simulink model "parallel"  (R2015b)
settings: Solver=FixedStepDiscrete  SolverMode=SingleTasking  StartTime=0.0  StopTime=600e-6  RelTol=1e-3
values from neighbouring files (symbols this model uses):
  b = ['00';'02';'04';'06';'08';'0a';'0c';'0e';'10';'12';'14';'16';'18';'1a';'1c';'1e';'20';'22';'24';'26';'28';'2a';'2c';'2e';'30';'32';'34';'36';'38';'3a';'3c';'3e';'40';'42';'44';'46';'48';'4a';'4c';'4e';'50';'52';'54';'56';'58';'5a';'5c';'5e';'60';'62';'64';'66';'68';'6a';'6c';'6e';'70';'72';'74';'76';'78';'7a';'7c';'7e';'80';'82';'84';'86';'88';'8a';'8c';'8e';'90';'92';'94';'96';'98';'9a';'9c';'9e' ...(+881 chars)    [parallelpipe_tb.m]
  input_sample_rate = 1.0E06    (= 1000000)    [parallelpipe_tb.m]
undefined symbols (not defined in the file or in its folder): a
libraries: shlslibv1 x6037
(part 2 of 40)

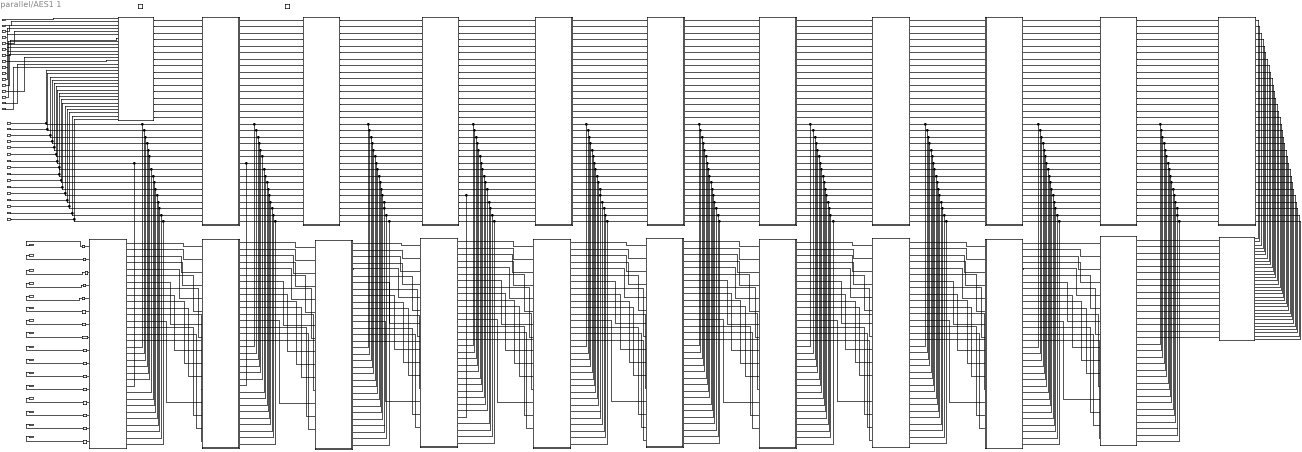
== system parallel/AES1 1 ==
  In1 : Inport
  In2 : Inport  Port=2
  In3 : Inport  Port=3
  In4 : Inport  Port=4
  In5 : Inport  Port=5
  In6 : Inport  Port=6
  In7 : Inport  Port=7
  In8 : Inport  Port=8
  In9 : Inport  Port=9
  In10 : Inport  Port=10
  In11 : Inport  Port=11
  In12 : Inport  Port=12
  In13 : Inport  Port=13
  In14 : Inport  Port=14
  In15 : Inport  Port=15
  In16 : Inport  Port=16
  In17 : Inport  Port=17
  In18 : Inport  Port=18
  In19 : Inport  Port=19
  In20 : Inport  Port=20
  In21 : Inport  Port=21
  In22 : Inport  Port=22
  In23 : Inport  Port=23
  In24 : Inport  Port=24
  In25 : Inport  Port=25
  In26 : Inport  Port=26
  In27 : Inport  Port=27
  In28 : Inport  Port=28
  In29 : Inport  Port=29
  In30 : Inport  Port=30
  In31 : Inport  Port=31
  In32 : Inport  Port=32
  Port Out{32..47} (16 alike) : shlslibv1/Ports & Subsystems/Port Out  syn_capture=on  syn_register=on  synBlockType=port  synLatency=1  synBlockId=1
  Round1 : Subsystem
  Round10 : Subsystem
  Round11 : Subsystem
  Round12 : Subsystem
  Round13 : Subsystem
  Round14 : Subsystem
  Round15 : Subsystem
  Round16 : Subsystem
  Round17 : Subsystem
  Round18 : Subsystem
  Round19 : Subsystem
  Round2 : Subsystem
  Round20 : Subsystem
  Round3 : Subsystem
  Round4 : Subsystem
  Round5 : Subsystem
  Round6 : Subsystem
  Round7 : Subsystem
  Round8 : Subsystem
  Round9 : Subsystem
  SHLSTool1 : shlslibv1/SHLSTool  synBlockType=tool  syn_dsp_mode=FPGA
  Subsystem : Subsystem
  Subsystem2 : Subsystem
  Test Vector Capture : shlslibv1/Ports & Subsystems/Test Vector Capture  syn_capture_mode=on
  Out1 : Outport
  Out2 : Outport  Port=2
  Out3 : Outport  Port=3
  Out4 : Outport  Port=4
  Out5 : Outport  Port=5
  Out6 : Outport  Port=6
  Out7 : Outport  Port=7
  Out8 : Outport  Port=8
  Out9 : Outport  Port=9
  Out10 : Outport  Port=10
  Out11 : Outport  Port=11
  Out12 : Outport  Port=12
  Out13 : Outport  Port=13
  Out14 : Outport  Port=14
  Out15 : Outport  Port=15
  Out16 : Outport  Port=16
  wires:
  Round1/1(Out1) -> Round2/1(In1)
  Round1/2(Out2) -> Round2/2(In2)
  Round1/3(Out3) -> Round2/3(In3)
  Round1/4(Out4) -> Round2/4(In4)
  Round1/5(Out5) -> Round2/5(In5)
  Round1/6(Out6) -> Round2/6(In6)
  Round1/7(Out7) -> Round2/7(In7)
  Round1/8(Out8) -> Round2/8(In8)
  Round1/9(Out9) -> Round2/9(In9)
  Round1/10(Out10) -> Round2/10(In10)
  Round1/11(Out11) -> Round2/11(In11)
  Round1/12(Out12) -> Round2/12(In12)
  Round1/13(Out13) -> Round2/13(In13)
  Round1/14(Out14) -> Round2/14(In14)
  Round1/15(Out15) -> Round2/15(In15)
  Round1/16(Out16) -> Round2/16(In16)
  Round2/2(Out2) -> Round4/2(In2)
  Round2/3(Out3) -> Round4/3(In3)
  Round2/4(Out4) -> Round4/4(In4)
  Round2/5(Out5) -> Round4/5(In5)
  Round2/6(Out6) -> Round4/6(In6)
  Round2/7(Out7) -> Round4/7(In7)
  Round2/8(Out8) -> Round4/8(In8)
  Round2/9(Out9) -> Round4/9(In9)
  Round2/10(Out10) -> Round4/10(In10)
  Round2/11(Out11) -> Round4/11(In11)
  Round2/12(Out12) -> Round4/12(In12)
  Round2/13(Out13) -> Round4/13(In13)
  Round2/14(Out14) -> Round4/14(In14)
  Round2/15(Out15) -> Round4/15(In15)
  Round2/16(Out16) -> Round4/16(In16)
  Round2/1(Out1) -> Round4/1(In1)
  Round4/1(Out1) -> Round5/1(In1)
  Round4/2(Out2) -> Round5/2(In2)
  Round3/2(Out2) -> Round6/2(In2)
  Round4/3(Out3) -> Round5/3(In3)
  Round4/4(Out4) -> Round5/4(In4)
  Round4/5(Out5) -> Round5/5(In5)
  Round4/6(Out6) -> Round5/6(In6)
  Round4/7(Out7) -> Round5/7(In7)
  Round4/8(Out8) -> Round5/8(In8)
  Round4/9(Out9) -> Round5/9(In9)
  Round4/10(Out10) -> Round5/10(In10)
  Round4/11(Out11) -> Round5/11(In11)
  Round4/12(Out12) -> Round5/12(In12)
  Round4/13(Out13) -> Round5/13(In13)
  Round4/14(Out14) -> Round5/14(In14)
  Round4/15(Out15) -> Round5/15(In15)
  Round4/16(Out16) -> Round5/16(In16)
  Round5/2(Out2) -> Round3/2(In2)
  Round5/3(Out3) -> Round3/3(In3)
  Round5/4(Out4) -> Round3/4(In4)
  Round5/5(Out5) -> Round3/5(In5)
  Round5/6(Out6) -> Round3/6(In6)
  Round5/7(Out7) -> Round3/7(In7)
  Round5/8(Out8) -> Round3/8(In8)
  Round5/9(Out9) -> Round3/9(In9)
  Round5/10(Out10) -> Round3/10(In10)
  Round5/11(Out11) -> Round3/11(In11)
  Round5/12(Out12) -> Round3/12(In12)
  Round5/13(Out13) -> Round3/13(In13)
  Round5/14(Out14) -> Round3/14(In14)
  Round5/15(Out15) -> Round3/15(In15)
  Round5/16(Out16) -> Round3/16(In16)
  Round5/1(Out1) -> Round3/1(In1)
  Round3/1(Out1) -> Round6/1(In1)
  Round9/3(Out3) -> Round10/3(In3)
  Round9/2(Out2) -> Round10/2(In2)
  Round3/3(Out3) -> Round6/3(In3)
  Round3/4(Out4) -> Round6/4(In4)
  Round3/5(Out5) -> Round6/5(In5)
  Round3/6(Out6) -> Round6/6(In6)
  Round3/7(Out7) -> Round6/7(In7)
  Round3/8(Out8) -> Round6/8(In8)
  Round3/9(Out9) -> Round6/9(In9)
  Round3/10(Out10) -> Round6/10(In10)
  Round3/11(Out11) -> Round6/11(In11)
  Round3/12(Out12) -> Round6/12(In12)
  Round3/13(Out13) -> Round6/13(In13)
  Round3/14(Out14) -> Round6/14(In14)
  Round3/15(Out15) -> Round6/15(In15)
  Round3/16(Out16) -> Round6/16(In16)
  Round6/1(Out1) -> Round7/1(In1)
  Round6/2(Out2) -> Round7/2(In2)
  Round6/3(Out3) -> Round7/3(In3)
  Round6/4(Out4) -> Round7/4(In4)
  Round6/5(Out5) -> Round7/5(In5)
  Round6/6(Out6) -> Round7/6(In6)
  Round6/7(Out7) -> Round7/7(In7)
  Round6/8(Out8) -> Round7/8(In8)
  Round6/9(Out9) -> Round7/9(In9)
  Round6/10(Out10) -> Round7/10(In10)
  Round6/11(Out11) -> Round7/11(In11)
  Round6/12(Out12) -> Round7/12(In12)
  Round6/13(Out13) -> Round7/13(In13)
  Round6/14(Out14) -> Round7/14(In14)
  Round6/15(Out15) -> Round7/15(In15)
  Round6/16(Out16) -> Round7/16(In16)
  Round7/1(Out1) -> Round8/1(In1)
  Round7/2(Out2) -> Round8/2(In2)
  Round7/3(Out3) -> Round8/3(In3)
  Round7/4(Out4) -> Round8/4(In4)
  Round7/5(Out5) -> Round8/5(In5)
  Round7/6(Out6) -> Round8/6(In6)
  Round7/7(Out7) -> Round8/7(In7)
  Round7/8(Out8) -> Round8/8(In8)
  Round7/9(Out9) -> Round8/9(In9)
  Round7/10(Out10) -> Round8/10(In10)
  Round7/11(Out11) -> Round8/11(In11)
  Round7/12(Out12) -> Round8/12(In12)
  Round7/13(Out13) -> Round8/13(In13)
  Round7/14(Out14) -> Round8/14(In14)
  Round7/15(Out15) -> Round8/15(In15)
  Round7/16(Out16) -> Round8/16(In16)
  Round8/1(Out1) -> Round9/1(In1)
  Round8/2(Out2) -> Round9/2(In2)
  Round8/3(Out3) -> Round9/3(In3)
  Round8/4(Out4) -> Round9/4(In4)
  Round8/5(Out5) -> Round9/5(In5)
  Round8/6(Out6) -> Round9/6(In6)
  Round8/7(Out7) -> Round9/7(In7)
  Round8/8(Out8) -> Round9/8(In8)
  Round8/9(Out9) -> Round9/9(In9)
  Round8/10(Out10) -> Round9/10(In10)
  Round8/11(Out11) -> Round9/11(In11)
  Round8/12(Out12) -> Round9/12(In12)
  Round8/13(Out13) -> Round9/13(In13)
  Round8/14(Out14) -> Round9/14(In14)
  Round8/15(Out15) -> Round9/15(In15)
  Round8/16(Out16) -> Round9/16(In16)
  Round9/1(Out1) -> Round10/1(In1)
  Round9/21(Out21) -> Round13/21(In21), Round10/21(In21)
  Round9/19(Out19) -> Round13/19(In19), Round10/19(In19)
  Round9/4(Out4) -> Round10/4(In4)
  Round9/5(Out5) -> Round10/5(In5)
  Round9/6(Out6) -> Round10/6(In6)
  Round9/7(Out7) -> Round10/7(In7)
  Round9/8(Out8) -> Round10/8(In8)
  Round9/9(Out9) -> Round10/9(In9)
  Round9/10(Out10) -> Round10/10(In10)
  Round9/11(Out11) -> Round10/11(In11)
  Round9/12(Out12) -> Round10/12(In12)
  Round9/13(Out13) -> Round10/13(In13)
  Round9/14(Out14) -> Round10/14(In14)
  Round9/15(Out15) -> Round10/15(In15)
  Round9/16(Out16) -> Round10/16(In16)
  Subsystem/1(Out1) -> Round1/1(In1)
  Subsystem/2(Out2) -> Round1/2(In2)
  Subsystem/3(Out3) -> Round1/3(In3)
  Subsystem/4(Out4) -> Round1/4(In4)
  Subsystem/5(Out5) -> Round1/5(In5)
  Subsystem/6(Out6) -> Round1/6(In6)
  Subsystem/7(Out7) -> Round1/7(In7)
  Subsystem/8(Out8) -> Round1/8(In8)
  Subsystem/9(Out9) -> Round1/9(In9)
  Subsystem/10(Out10) -> Round1/10(In10)
  Subsystem/11(Out11) -> Round1/11(In11)
  Subsystem/12(Out12) -> Round1/12(In12)
  Subsystem/13(Out13) -> Round1/13(In13)
  Subsystem/14(Out14) -> Round1/14(In14)
  Subsystem/15(Out15) -> Round1/15(In15)
  Subsystem/16(Out16) -> Round1/16(In16)
  In1/1 -> Subsystem/1(In1)
  In2/1 -> Subsystem/2(In2)
  In3/1 -> Subsystem/3(In3)
  In4/1 -> Subsystem/4(In4)
  In5/1 -> Subsystem/5(In5)
  In6/1 -> Subsystem/6(In6)
  In7/1 -> Subsystem/7(In7)
  In8/1 -> Subsystem/8(In8)
  In9/1 -> Subsystem/9(In9)
  In10/1 -> Subsystem/10(In10)
  In11/1 -> Subsystem/11(In11)
  In12/1 -> Subsystem/12(In12)
  In13/1 -> Subsystem/13(In13)
  In14/1 -> Subsystem/14(In14)
  In15/1 -> Subsystem/15(In15)
  In16/1 -> Subsystem/16(In16)
  Round10/11(Out11) -> Subsystem2/11(In11)
  Round10/13(Out13) -> Subsystem2/13(In13)
  Round10/15(Out15) -> Subsystem2/15(In15)
  Round10/17(Out17) -> Subsystem2/17(In17)
  Round10/19(Out19) -> Subsystem2/19(In19)
  Round10/21(Out21) -> Subsystem2/21(In21)
  Round10/23(Out23) -> Subsystem2/23(In23)
  Round10/27(Out27) -> Subsystem2/27(In27)
  Round10/29(Out29) -> Subsystem2/29(In29)
  Round10/25(Out25) -> Subsystem2/25(In25)
  Round10/2(Out2) -> Subsystem2/2(In2)
  Round10/12(Out12) -> Subsystem2/12(In12)
  Round10/14(Out14) -> Subsystem2/14(In14)
  Round10/16(Out16) -> Subsystem2/16(In16)
  Round10/18(Out18) -> Subsystem2/18(In18)
  Round10/20(Out20) -> Subsystem2/20(In20)
  Round10/22(Out22) -> Subsystem2/22(In22)
  Round10/24(Out24) -> Subsystem2/24(In24)
  Round10/28(Out28) -> Subsystem2/28(In28)
  Round10/30(Out30) -> Subsystem2/30(In30)
  Round10/26(Out26) -> Subsystem2/26(In26)
  Round10/1(Out1) -> Subsystem2/1(In1)
  Round10/3(Out3) -> Subsystem2/3(In3)
  Round10/4(Out4) -> Subsystem2/4(In4)
  Round10/5(Out5) -> Subsystem2/5(In5)
  Round10/6(Out6) -> Subsystem2/6(In6)
  Round10/7(Out7) -> Subsystem2/7(In7)
  Round10/8(Out8) -> Subsystem2/8(In8)
  Round10/9(Out9) -> Subsystem2/9(In9)
  Round10/10(Out10) -> Subsystem2/10(In10)
  Round10/31(Out31) -> Subsystem2/31(In31)
  Round10/32(Out32) -> Subsystem2/32(In32)
  Subsystem2/1(Out1) -> Round13/1(In1)
  Subsystem2/2(Out2) -> Round13/2(In2)
  Subsystem2/3(Out3) -> Round13/3(In3)
  Subsystem2/4(Out4) -> Round13/4(In4)
  Subsystem2/5(Out5) -> Round13/5(In5)
  Subsystem2/6(Out6) -> Round13/6(In6)
  Subsystem2/7(Out7) -> Round13/7(In7)
  Subsystem2/8(Out8) -> Round13/8(In8)
  Subsystem2/9(Out9) -> Round13/9(In9)
  Subsystem2/10(Out10) -> Round13/10(In10)
  Subsystem2/11(Out11) -> Round13/11(In11)
  Subsystem2/12(Out12) -> Round13/12(In12)
  Subsystem2/13(Out13) -> Round13/13(In13)
  Subsystem2/14(Out14) -> Round13/14(In14)
  Subsystem2/15(Out15) -> Round13/15(In15)
  Subsystem2/16(Out16) -> Round13/16(In16)
  Round9/17(Out17) -> Round13/17(In17), Round10/17(In17)
  Round1/17(Out17) -> Round19/17(In17), Round2/17(In17)
  Round1/19(Out19) -> Round19/19(In19), Round2/19(In19)
  Round1/21(Out21) -> Round19/21(In21), Round2/21(In21)
  Round1/23(Out23) -> Round2/23(In23), Round19/23(In23)
  Round9/23(Out23) -> Round13/23(In23), Round10/23(In23)
  Round9/27(Out27) -> Round13/27(In27), Round10/27(In27)
  Round9/29(Out29) -> Round13/29(In29), Round10/29(In29)
  Round9/25(Out25) -> Round13/25(In25), Round10/25(In25)
  Round9/18(Out18) -> Round13/18(In18), Round10/18(In18)
  Round9/20(Out20) -> Round13/20(In20), Round10/20(In20)
  Round9/22(Out22) -> Round13/22(In22), Round10/22(In22)
  Round9/24(Out24) -> Round13/24(In24), Round10/24(In24)
  Round9/28(Out28) -> Round13/28(In28), Round10/28(In28)
  Round9/30(Out30) -> Round13/30(In30), Round10/30(In30)
  Round9/26(Out26) -> Round13/26(In26), Round10/26(In26)
  Round9/31(Out31) -> Round13/31(In31), Round10/31(In31)
  Round9/32(Out32) -> Round13/32(In32), Round10/32(In32)
  Port Out32/1 -> Out1/1
  Port Out33/1 -> Out2/1
  Port Out36/1 -> Out3/1
  Port Out42/1 -> Out4/1
  Port Out43/1 -> Out5/1
  Port Out44/1 -> Out6/1
  Port Out45/1 -> Out7/1
  Port Out46/1 -> Out8/1
  Port Out47/1 -> Out10/1
  Port Out34/1 -> Out11/1
  Port Out35/1 -> Out12/1
  Port Out37/1 -> Out13/1
  Port Out38/1 -> Out14/1
  Port Out39/1 -> Out15/1
  Port Out40/1 -> Out16/1
  Round13/1(Out1) -> Round11/1(In1)
  Round8/17(Out17) -> Round11/17(In17), Round9/17(In17)
  Round8/19(Out19) -> Round11/19(In19), Round9/19(In19)
  Round8/21(Out21) -> Round11/21(In21), Round9/21(In21)
  Round8/23(Out23) -> Round11/23(In23), Round9/23(In23)
  Round8/27(Out27) -> Round11/27(In27), Round9/27(In27)
  Round8/29(Out29) -> Round11/29(In29), Round9/29(In29)
  Round8/25(Out25) -> Round11/25(In25), Round9/25(In25)
  Round8/18(Out18) -> Round11/18(In18), Round9/18(In18)
  Round8/20(Out20) -> Round11/20(In20), Round9/20(In20)
  Round8/22(Out22) -> Round11/22(In22), Round9/22(In22)
  Round8/24(Out24) -> Round11/24(In24), Round9/24(In24)
  Round8/28(Out28) -> Round11/28(In28), Round9/28(In28)
  Round8/30(Out30) -> Round11/30(In30), Round9/30(In30)
  Round8/26(Out26) -> Round11/26(In26), Round9/26(In26)
  Round8/31(Out31) -> Round11/31(In31), Round9/31(In31)
  Round8/32(Out32) -> Round11/32(In32), Round9/32(In32)
  Round13/2(Out2) -> Round11/2(In2)
  Round13/3(Out3) -> Round11/3(In3)
  Round13/4(Out4) -> Round11/4(In4)
  Round13/5(Out5) -> Round11/5(In5)
  Round13/6(Out6) -> Round11/6(In6)
  Round13/7(Out7) -> Round11/7(In7)
  Round13/8(Out8) -> Round11/8(In8)
  Round13/9(Out9) -> Round11/9(In9)
  Round13/10(Out10) -> Round11/10(In10)
  Round13/11(Out11) -> Round11/11(In11)
  Round13/12(Out12) -> Round11/12(In12)
  Round13/13(Out13) -> Round11/13(In13)
  Round13/14(Out14) -> Round11/14(In14)
  Round13/15(Out15) -> Round11/15(In15)
  Round13/16(Out16) -> Round11/16(In16)
  Port Out41/1 -> Out9/1
  Round11/1(Out1) -> Round12/1(In1)
  Round7/17(Out17) -> Round12/17(In17), Round8/17(In17)
  Round7/19(Out19) -> Round12/19(In19), Round8/19(In19)
  Round7/21(Out21) -> Round12/21(In21), Round8/21(In21)
  Round7/23(Out23) -> Round12/23(In23), Round8/23(In23)
  Round7/27(Out27) -> Round12/27(In27), Round8/27(In27)
  Round7/29(Out29) -> Round12/29(In29), Round8/29(In29)
  Round7/25(Out25) -> Round12/25(In25), Round8/25(In25)
  Round7/18(Out18) -> Round12/18(In18), Round8/18(In18)
  Round7/20(Out20) -> Round12/20(In20), Round8/20(In20)
  Round7/22(Out22) -> Round12/22(In22), Round8/22(In22)
  Round7/24(Out24) -> Round12/24(In24), Round8/24(In24)
  Round7/28(Out28) -> Round12/28(In28), Round8/28(In28)
  Round7/30(Out30) -> Round12/30(In30), Round8/30(In30)
  Round7/26(Out26) -> Round12/26(In26), Round8/26(In26)
  Round7/31(Out31) -> Round12/31(In31), Round8/31(In31)
  Round7/32(Out32) -> Round12/32(In32), Round8/32(In32)
  Round11/2(Out2) -> Round12/2(In2)
  Round11/3(Out3) -> Round12/3(In3)
  Round11/4(Out4) -> Round12/4(In4)
  Round11/5(Out5) -> Round12/5(In5)
  Round11/6(Out6) -> Round12/6(In6)
  Round11/7(Out7) -> Round12/7(In7)
  Round11/8(Out8) -> Round12/8(In8)
  Round11/9(Out9) -> Round12/9(In9)
  Round11/10(Out10) -> Round12/10(In10)
  Round11/11(Out11) -> Round12/11(In11)
  Round11/12(Out12) -> Round12/12(In12)
  Round11/13(Out13) -> Round12/13(In13)
  Round11/14(Out14) -> Round12/14(In14)
  Round11/15(Out15) -> Round12/15(In15)
  Round11/16(Out16) -> Round12/16(In16)
  Round12/1(Out1) -> Round14/1(In1)
  Round6/17(Out17) -> Round14/17(In17), Round7/17(In17)
  Round6/19(Out19) -> Round14/19(In19), Round7/19(In19)
  Round6/21(Out21) -> Round14/21(In21), Round7/21(In21)
  Round6/23(Out23) -> Round14/23(In23), Round7/23(In23)
  Round6/27(Out27) -> Round14/27(In27), Round7/27(In27)
  Round6/29(Out29) -> Round14/29(In29), Round7/29(In29)
  Round6/25(Out25) -> Round14/25(In25), Round7/25(In25)
  Round6/18(Out18) -> Round14/18(In18), Round7/18(In18)
  Round6/20(Out20) -> Round14/20(In20), Round7/20(In20)
  Round6/22(Out22) -> Round14/22(In22), Round7/22(In22)
  Round6/24(Out24) -> Round14/24(In24), Round7/24(In24)
  Round6/28(Out28) -> Round14/28(In28), Round7/28(In28)
  Round6/30(Out30) -> Round14/30(In30), Round7/30(In30)
  Round6/26(Out26) -> Round14/26(In26), Round7/26(In26)
  Round6/31(Out31) -> Round14/31(In31), Round7/31(In31)
  Round6/32(Out32) -> Round14/32(In32), Round7/32(In32)
  Round12/2(Out2) -> Round14/2(In2)
  Round12/3(Out3) -> Round14/3(In3)
  Round12/4(Out4) -> Round14/4(In4)
  Round12/5(Out5) -> Round14/5(In5)
  Round12/6(Out6) -> Round14/6(In6)
  Round12/7(Out7) -> Round14/7(In7)
  Round12/8(Out8) -> Round14/8(In8)
  Round12/9(Out9) -> Round14/9(In9)
  Round12/10(Out10) -> Round14/10(In10)
  Round12/11(Out11) -> Round14/11(In11)
  Round12/12(Out12) -> Round14/12(In12)
  Round12/13(Out13) -> Round14/13(In13)
  Round12/14(Out14) -> Round14/14(In14)
  Round12/15(Out15) -> Round14/15(In15)
  Round12/16(Out16) -> Round14/16(In16)
  Round14/1(Out1) -> Round15/1(In1)
  Round3/17(Out17) -> Round15/17(In17), Round6/17(In17)
  Round3/19(Out19) -> Round15/19(In19), Round6/19(In19)
  Round3/21(Out21) -> Round15/21(In21), Round6/21(In21)
  Round3/23(Out23) -> Round15/23(In23), Round6/23(In23)
  Round3/27(Out27) -> Round15/27(In27), Round6/27(In27)
  Round3/29(Out29) -> Round15/29(In29), Round6/29(In29)
  Round3/25(Out25) -> Round15/25(In25), Round6/25(In25)
  Round3/18(Out18) -> Round15/18(In18), Round6/18(In18)
  Round3/20(Out20) -> Round15/20(In20), Round6/20(In20)
  Round3/22(Out22) -> Round15/22(In22), Round6/22(In22)
  Round3/24(Out24) -> Round15/24(In24), Round6/24(In24)
  Round3/28(Out28) -> Round15/28(In28), Round6/28(In28)
  Round3/30(Out30) -> Round15/30(In30), Round6/30(In30)
  Round3/26(Out26) -> Round15/26(In26), Round6/26(In26)
  Round3/31(Out31) -> Round15/31(In31), Round6/31(In31)
  Round3/32(Out32) -> Round15/32(In32), Round6/32(In32)
  Round14/2(Out2) -> Round15/2(In2)
  Round14/3(Out3) -> Round15/3(In3)
  Round14/4(Out4) -> Round15/4(In4)
  Round14/5(Out5) -> Round15/5(In5)
  Round14/6(Out6) -> Round15/6(In6)
  Round14/7(Out7) -> Round15/7(In7)
  Round14/8(Out8) -> Round15/8(In8)
  Round14/9(Out9) -> Round15/9(In9)
  Round14/10(Out10) -> Round15/10(In10)
  Round14/11(Out11) -> Round15/11(In11)
  Round14/12(Out12) -> Round15/12(In12)
  Round14/13(Out13) -> Round15/13(In13)
  Round14/14(Out14) -> Round15/14(In14)
  Round14/15(Out15) -> Round15/15(In15)
  Round14/16(Out16) -> Round15/16(In16)
  Round15/1(Out1) -> Round16/1(In1)
  Round5/17(Out17) -> Round16/17(In17), Round3/17(In17)
  Round5/19(Out19) -> Round16/19(In19), Round3/19(In19)
  Round5/21(Out21) -> Round16/21(In21), Round3/21(In21)
  Round5/23(Out23) -> Round16/23(In23), Round3/23(In23)
  Round5/27(Out27) -> Round16/27(In27), Round3/27(In27)
  Round5/29(Out29) -> Round16/29(In29), Round3/29(In29)
  Round5/25(Out25) -> Round16/25(In25), Round3/25(In25)
  Round5/18(Out18) -> Round16/18(In18), Round3/18(In18)
  Round5/20(Out20) -> Round16/20(In20), Round3/20(In20)
  Round5/22(Out22) -> Round16/22(In22), Round3/22(In22)
  Round5/24(Out24) -> Round16/24(In24), Round3/24(In24)
  Round5/28(Out28) -> Round16/28(In28), Round3/28(In28)
  Round5/30(Out30) -> Round16/30(In30), Round3/30(In30)
  Round5/26(Out26) -> Round16/26(In26), Round3/26(In26)
  Round5/31(Out31) -> Round16/31(In31), Round3/31(In31)
  Round5/32(Out32) -> Round16/32(In32), Round3/32(In32)
  Round15/2(Out2) -> Round16/2(In2)
  Round15/3(Out3) -> Round16/3(In3)
  Round15/4(Out4) -> Round16/4(In4)
  Round15/5(Out5) -> Round16/5(In5)
  Round15/6(Out6) -> Round16/6(In6)
  Round15/7(Out7) -> Round16/7(In7)
  Round15/8(Out8) -> Round16/8(In8)
  Round15/9(Out9) -> Round16/9(In9)
  Round15/10(Out10) -> Round16/10(In10)
  Round15/11(Out11) -> Round16/11(In11)
  Round15/12(Out12) -> Round16/12(In12)
  Round15/13(Out13) -> Round16/13(In13)
  Round15/14(Out14) -> Round16/14(In14)
  Round15/15(Out15) -> Round16/15(In15)
  Round15/16(Out16) -> Round16/16(In16)
  Round16/1(Out1) -> Round17/1(In1)
  Round4/17(Out17) -> Round17/17(In17), Round5/17(In17)
  Round4/19(Out19) -> Round17/19(In19), Round5/19(In19)
  Round4/21(Out21) -> Round17/21(In21), Round5/21(In21)
  Round4/23(Out23) -> Round17/23(In23), Round5/23(In23)
  Round4/27(Out27) -> Round17/27(In27), Round5/27(In27)
  Round4/29(Out29) -> Round17/29(In29), Round5/29(In29)
  Round4/25(Out25) -> Round17/25(In25), Round5/25(In25)
  Round4/18(Out18) -> Round17/18(In18), Round5/18(In18)
  Round4/20(Out20) -> Round17/20(In20), Round5/20(In20)
  Round4/22(Out22) -> Round17/22(In22), Round5/22(In22)
  Round4/24(Out24) -> Round17/24(In24), Round5/24(In24)
  Round4/28(Out28) -> Round5/28(In28), Round17/28(In28)
  Round4/30(Out30) -> Round17/30(In30), Round5/30(In30)
  Round4/26(Out26) -> Round17/26(In26), Round5/26(In26)
  Round4/31(Out31) -> Round17/31(In31), Round5/31(In31)
  Round4/32(Out32) -> Round17/32(In32), Round5/32(In32)
  Round16/2(Out2) -> Round17/2(In2)
  Round16/3(Out3) -> Round17/3(In3)
  Round16/4(Out4) -> Round17/4(In4)
  Round16/5(Out5) -> Round17/5(In5)
  Round16/6(Out6) -> Round17/6(In6)
  Round16/7(Out7) -> Round17/7(In7)
  Round16/8(Out8) -> Round17/8(In8)
  Round16/9(Out9) -> Round17/9(In9)
  Round16/10(Out10) -> Round17/10(In10)
  Round16/11(Out11) -> Round17/11(In11)
  Round16/12(Out12) -> Round17/12(In12)
  Round16/13(Out13) -> Round17/13(In13)
  Round16/14(Out14) -> Round17/14(In14)
  Round16/15(Out15) -> Round17/15(In15)
  Round16/16(Out16) -> Round17/16(In16)
  Round17/1(Out1) -> Round18/1(In1)
  Round2/17(Out17) -> Round18/17(In17), Round4/17(In17)
  Round2/19(Out19) -> Round18/19(In19), Round4/19(In19)
  Round2/21(Out21) -> Round18/21(In21), Round4/21(In21)
  Round2/23(Out23) -> Round18/23(In23), Round4/23(In23)
  Round2/27(Out27) -> Round18/27(In27), Round4/27(In27)
  Round2/29(Out29) -> Round18/29(In29), Round4/29(In29)
  Round2/25(Out25) -> Round18/25(In25), Round4/25(In25)
  Round2/18(Out18) -> Round18/18(In18), Round4/18(In18)
  Round2/20(Out20) -> Round18/20(In20), Round4/20(In20)
  Round2/22(Out22) -> Round18/22(In22), Round4/22(In22)
  Round2/24(Out24) -> Round18/24(In24), Round4/24(In24)
  Round2/28(Out28) -> Round18/28(In28), Round4/28(In28)
  Round2/30(Out30) -> Round4/30(In30), Round18/30(In30)
  Round2/26(Out26) -> Round18/26(In26), Round4/26(In26)
  Round2/31(Out31) -> Round18/31(In31), Round4/31(In31)
  Round2/32(Out32) -> Round18/32(In32), Round4/32(In32)
  Round17/2(Out2) -> Round18/2(In2)
  Round17/3(Out3) -> Round18/3(In3)
  Round17/4(Out4) -> Round18/4(In4)
  Round17/5(Out5) -> Round18/5(In5)
  Round17/6(Out6) -> Round18/6(In6)
  Round17/7(Out7) -> Round18/7(In7)
  Round17/8(Out8) -> Round18/8(In8)
  Round17/9(Out9) -> Round18/9(In9)
  Round17/10(Out10) -> Round18/10(In10)
  Round17/11(Out11) -> Round18/11(In11)
  Round17/12(Out12) -> Round18/12(In12)
  Round17/13(Out13) -> Round18/13(In13)
  Round17/14(Out14) -> Round18/14(In14)
  Round17/15(Out15) -> Round18/15(In15)
  Round17/16(Out16) -> Round18/16(In16)
  Round18/1(Out1) -> Round19/1(In1)
  Round1/27(Out27) -> Round19/27(In27), Round2/27(In27)
  Round1/29(Out29) -> Round19/29(In29), Round2/29(In29)
  Round1/25(Out25) -> Round19/25(In25), Round2/25(In25)
  Round1/18(Out18) -> Round19/18(In18), Round2/18(In18)
  Round1/20(Out20) -> Round19/20(In20), Round2/20(In20)
  Round1/22(Out22) -> Round19/22(In22), Round2/22(In22)
  Round1/24(Out24) -> Round19/24(In24), Round2/24(In24)
  Round1/28(Out28) -> Round19/28(In28), Round2/28(In28)
  Round1/30(Out30) -> Round19/30(In30), Round2/30(In30)
  Round1/26(Out26) -> Round19/26(In26), Round2/26(In26)
  Round1/31(Out31) -> Round19/31(In31), Round2/31(In31)
  Round1/32(Out32) -> Round19/32(In32), Round2/32(In32)
  Round18/2(Out2) -> Round19/2(In2)
  Round18/3(Out3) -> Round19/3(In3)
  Round18/4(Out4) -> Round19/4(In4)
  Round18/5(Out5) -> Round19/5(In5)
  Round18/6(Out6) -> Round19/6(In6)
  Round18/7(Out7) -> Round19/7(In7)
  Round18/8(Out8) -> Round19/8(In8)
  Round18/9(Out9) -> Round19/9(In9)
  Round18/10(Out10) -> Round19/10(In10)
  Round18/11(Out11) -> Round19/11(In11)
  Round18/12(Out12) -> Round19/12(In12)
  Round18/13(Out13) -> Round19/13(In13)
  Round18/14(Out14) -> Round19/14(In14)
  Round18/15(Out15) -> Round19/15(In15)
  Round18/16(Out16) -> Round19/16(In16)
  Round19/1(Out1) -> Round20/1(In1)
  In17/1 -> Round20/17(In17), Round1/17(In17), Subsystem/17(In17)
  In19/1 -> Subsystem/19(In19), Round20/19(In19), Round1/19(In19)
  In21/1 -> Subsystem/21(In21), Round20/21(In21), Round1/21(In21)
  In23/1 -> Subsystem/23(In23), Round20/23(In23), Round1/23(In23)
  In27/1 -> Subsystem/27(In27), Round20/27(In27), Round1/27(In27)
  In29/1 -> Subsystem/29(In29), Round20/29(In29), Round1/29(In29)
  In25/1 -> Subsystem/25(In25), Round20/25(In25), Round1/25(In25)
  In18/1 -> Subsystem/18(In18), Round20/18(In18), Round1/18(In18)
  In20/1 -> Subsystem/20(In20), Round20/20(In20), Round1/20(In20)
  In22/1 -> Subsystem/22(In22), Round20/22(In22), Round1/22(In22)
  In24/1 -> Subsystem/24(In24), Round20/24(In24), Round1/24(In24)
  In28/1 -> Subsystem/28(In28), Round20/28(In28), Round1/28(In28)
  In30/1 -> Subsystem/30(In30), Round20/30(In30), Round1/30(In30)
  In26/1 -> Subsystem/26(In26), Round20/26(In26), Round1/26(In26)
  In31/1 -> Subsystem/31(In31), Round20/31(In31), Round1/31(In31)
  In32/1 -> Subsystem/32(In32), Round20/32(In32), Round1/32(In32)
  Round19/2(Out2) -> Round20/2(In2)
  Round19/3(Out3) -> Round20/3(In3)
  Round19/4(Out4) -> Round20/4(In4)
  Round19/5(Out5) -> Round20/5(In5)
  Round19/6(Out6) -> Round20/6(In6)
  Round19/7(Out7) -> Round20/7(In7)
  Round19/8(Out8) -> Round20/8(In8)
  Round19/9(Out9) -> Round20/9(In9)
  Round19/10(Out10) -> Round20/10(In10)
  Round19/11(Out11) -> Round20/11(In11)
  Round19/12(Out12) -> Round20/12(In12)
  Round19/13(Out13) -> Round20/13(In13)
  Round19/14(Out14) -> Round20/14(In14)
  Round19/15(Out15) -> Round20/15(In15)
  Round19/16(Out16) -> Round20/16(In16)
  Round20/1(Out1) -> Port Out32/1
  Round20/2(Out2) -> Port Out33/1
  Round20/3(Out3) -> Port Out36/1
  Round20/4(Out4) -> Port Out42/1
  Round20/5(Out5) -> Port Out43/1
  Round20/6(Out6) -> Port Out44/1
  Round20/7(Out7) -> Port Out45/1
  Round20/8(Out8) -> Port Out46/1
  Round20/9(Out9) -> Port Out41/1
  Round20/10(Out10) -> Port Out47/1
  Round20/11(Out11) -> Port Out34/1
  Round20/12(Out12) -> Port Out35/1
  Round20/13(Out13) -> Port Out37/1
  Round20/14(Out14) -> Port Out38/1
  Round20/15(Out15) -> Port Out39/1
  Round20/16(Out16) -> Port Out40/1

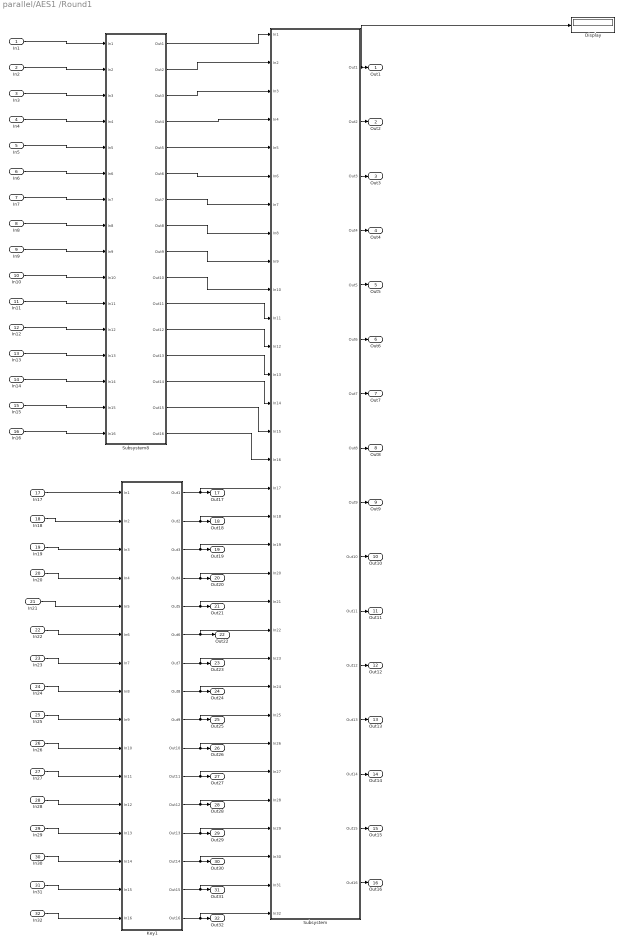
== system parallel/AES1 /Round1 ==
  In1 : Inport
  In2 : Inport  Port=2
  In3 : Inport  Port=3
  In4 : Inport  Port=4
  In5 : Inport  Port=5
  In6 : Inport  Port=6
  In7 : Inport  Port=7
  In8 : Inport  Port=8
  In9 : Inport  Port=9
  In10 : Inport  Port=10
  In11 : Inport  Port=11
  In12 : Inport  Port=12
  In13 : Inport  Port=13
  In14 : Inport  Port=14
  In15 : Inport  Port=15
  In16 : Inport  Port=16
  In17 : Inport  Port=17
  In18 : Inport  Port=18
  In19 : Inport  Port=19
  In20 : Inport  Port=20
  In21 : Inport  Port=21
  In22 : Inport  Port=22
  In23 : Inport  Port=23
  In24 : Inport  Port=24
  In25 : Inport  Port=25
  In26 : Inport  Port=26
  In27 : Inport  Port=27
  In28 : Inport  Port=28
  In29 : Inport  Port=29
  In30 : Inport  Port=30
  In31 : Inport  Port=31
  In32 : Inport  Port=32
  Display : Display
      settings: Format=hex (Stored Integer)
  Key1 : Subsystem
  Subsystem : Subsystem
  Subsystem8 : Subsystem
  Out1 : Outport
  Out2 : Outport  Port=2
  Out3 : Outport  Port=3
  Out4 : Outport  Port=4
  Out5 : Outport  Port=5
  Out6 : Outport  Port=6
  Out7 : Outport  Port=7
  Out8 : Outport  Port=8
  Out9 : Outport  Port=9
  Out10 : Outport  Port=10
  Out11 : Outport  Port=11
  Out12 : Outport  Port=12
  Out13 : Outport  Port=13
  Out14 : Outport  Port=14
  Out15 : Outport  Port=15
  Out16 : Outport  Port=16
  Out17 : Outport  Port=17
  Out18 : Outport  Port=18
  Out19 : Outport  Port=19
  Out20 : Outport  Port=20
  Out21 : Outport  Port=21
  Out22 : Outport  Port=22
  Out23 : Outport  Port=23
  Out24 : Outport  Port=24
  Out25 : Outport  Port=25
  Out26 : Outport  Port=26
  Out27 : Outport  Port=27
  Out28 : Outport  Port=28
  Out29 : Outport  Port=29
  Out30 : Outport  Port=30
  Out31 : Outport  Port=31
  Out32 : Outport  Port=32
  wires:
  Subsystem/14(Out14) -> Out14/1
  Subsystem/6(Out6) -> Out6/1
  Subsystem/13(Out13) -> Out13/1
  Subsystem/10(Out10) -> Out10/1
  Subsystem/5(Out5) -> Out5/1
  Subsystem/7(Out7) -> Out7/1
  Subsystem/8(Out8) -> Out8/1
  Subsystem/3(Out3) -> Out3/1
  Subsystem/2(Out2) -> Out2/1
  Subsystem/16(Out16) -> Out16/1
  Subsystem/9(Out9) -> Out9/1
  Subsystem/12(Out12) -> Out12/1
  Subsystem/15(Out15) -> Out15/1
  Subsystem/4(Out4) -> Out4/1
  Subsystem/11(Out11) -> Out11/1
  In1/1 -> Subsystem8/1(In1)
  In3/1 -> Subsystem8/3(In3)
  In2/1 -> Subsystem8/2(In2)
  In4/1 -> Subsystem8/4(In4)
  In5/1 -> Subsystem8/5(In5)
  In7/1 -> Subsystem8/7(In7)
  In6/1 -> Subsystem8/6(In6)
  In9/1 -> Subsystem8/9(In9)
  In8/1 -> Subsystem8/8(In8)
  In12/1 -> Subsystem8/12(In12)
  In10/1 -> Subsystem8/10(In10)
  In11/1 -> Subsystem8/11(In11)
  In14/1 -> Subsystem8/14(In14)
  In13/1 -> Subsystem8/13(In13)
  In15/1 -> Subsystem8/15(In15)
  In16/1 -> Subsystem8/16(In16)
  Subsystem8/1(Out1) -> Subsystem/1(In1)
  Subsystem8/2(Out2) -> Subsystem/2(In2)
  Subsystem8/4(Out4) -> Subsystem/4(In4)
  Subsystem8/3(Out3) -> Subsystem/3(In3)
  Subsystem8/6(Out6) -> Subsystem/6(In6)
  Subsystem8/5(Out5) -> Subsystem/5(In5)
  Subsystem8/8(Out8) -> Subsystem/8(In8)
  Subsystem8/7(Out7) -> Subsystem/7(In7)
  Subsystem8/10(Out10) -> Subsystem/10(In10)
  Subsystem8/9(Out9) -> Subsystem/9(In9)
  Subsystem8/11(Out11) -> Subsystem/11(In11)
  Subsystem8/12(Out12) -> Subsystem/12(In12)
  Subsystem8/13(Out13) -> Subsystem/13(In13)
  Subsystem8/15(Out15) -> Subsystem/15(In15)
  Subsystem8/14(Out14) -> Subsystem/14(In14)
  Subsystem8/16(Out16) -> Subsystem/16(In16)
  In17/1 -> Key1/1(In1)
  In19/1 -> Key1/3(In3)
  In18/1 -> Key1/2(In2)
  In21/1 -> Key1/5(In5)
  In20/1 -> Key1/4(In4)
  In23/1 -> Key1/7(In7)
  In22/1 -> Key1/6(In6)
  In25/1 -> Key1/9(In9)
  In24/1 -> Key1/8(In8)
  In27/1 -> Key1/11(In11)
  In26/1 -> Key1/10(In10)
  In29/1 -> Key1/13(In13)
  In28/1 -> Key1/12(In12)
  In30/1 -> Key1/14(In14)
  In31/1 -> Key1/15(In15)
  In32/1 -> Key1/16(In16)
  Key1/14(Out14) -> Out30/1, Subsystem/30(In30)
  Key1/6(Out6) -> Out22/1, Subsystem/22(In22)
  Key1/13(Out13) -> Out29/1, Subsystem/29(In29)
  Key1/10(Out10) -> Out26/1, Subsystem/26(In26)
  Key1/5(Out5) -> Out21/1, Subsystem/21(In21)
  Key1/1(Out1) -> Out17/1, Subsystem/17(In17)
  Key1/7(Out7) -> Out23/1, Subsystem/23(In23)
  Key1/8(Out8) -> Out24/1, Subsystem/24(In24)
  Key1/3(Out3) -> Out19/1, Subsystem/19(In19)
  Key1/2(Out2) -> Out18/1, Subsystem/18(In18)
  Key1/16(Out16) -> Out32/1, Subsystem/32(In32)
  Key1/9(Out9) -> Out25/1, Subsystem/25(In25)
  Key1/12(Out12) -> Out28/1, Subsystem/28(In28)
  Key1/15(Out15) -> Out31/1, Subsystem/31(In31)
  Key1/4(Out4) -> Out20/1, Subsystem/20(In20)
  Key1/11(Out11) -> Out27/1, Subsystem/27(In27)
  Subsystem/1(Out1) -> Display/1, Out1/1

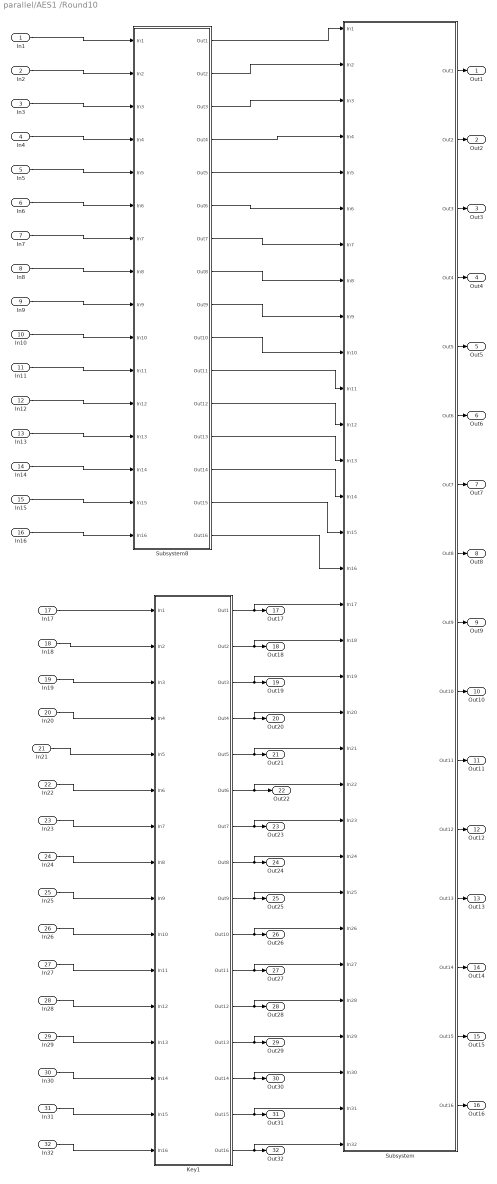
== system parallel/AES1 /Round10 ==
  In1 : Inport
  In2 : Inport  Port=2
  In3 : Inport  Port=3
  In4 : Inport  Port=4
  In5 : Inport  Port=5
  In6 : Inport  Port=6
  In7 : Inport  Port=7
  In8 : Inport  Port=8
  In9 : Inport  Port=9
  In10 : Inport  Port=10
  In11 : Inport  Port=11
  In12 : Inport  Port=12
  In13 : Inport  Port=13
  In14 : Inport  Port=14
  In15 : Inport  Port=15
  In16 : Inport  Port=16
  In17 : Inport  Port=17
  In18 : Inport  Port=18
  In19 : Inport  Port=19
  In20 : Inport  Port=20
  In21 : Inport  Port=21
  In22 : Inport  Port=22
  In23 : Inport  Port=23
  In24 : Inport  Port=24
  In25 : Inport  Port=25
  In26 : Inport  Port=26
  In27 : Inport  Port=27
  In28 : Inport  Port=28
  In29 : Inport  Port=29
  In30 : Inport  Port=30
  In31 : Inport  Port=31
  In32 : Inport  Port=32
  Key1 : Subsystem
  Subsystem : Subsystem
  Subsystem8 : Subsystem
  Out1 : Outport
  Out2 : Outport  Port=2
  Out3 : Outport  Port=3
  Out4 : Outport  Port=4
  Out5 : Outport  Port=5
  Out6 : Outport  Port=6
  Out7 : Outport  Port=7
  Out8 : Outport  Port=8
  Out9 : Outport  Port=9
  Out10 : Outport  Port=10
  Out11 : Outport  Port=11
  Out12 : Outport  Port=12
  Out13 : Outport  Port=13
  Out14 : Outport  Port=14
  Out15 : Outport  Port=15
  Out16 : Outport  Port=16
  Out17 : Outport  Port=17
  Out18 : Outport  Port=18
  Out19 : Outport  Port=19
  Out20 : Outport  Port=20
  Out21 : Outport  Port=21
  Out22 : Outport  Port=22
  Out23 : Outport  Port=23
  Out24 : Outport  Port=24
  Out25 : Outport  Port=25
  Out26 : Outport  Port=26
  Out27 : Outport  Port=27
  Out28 : Outport  Port=28
  Out29 : Outport  Port=29
  Out30 : Outport  Port=30
  Out31 : Outport  Port=31
  Out32 : Outport  Port=32
  wires:
  Subsystem/14(Out14) -> Out14/1
  Subsystem/6(Out6) -> Out6/1
  Subsystem/13(Out13) -> Out13/1
  Subsystem/10(Out10) -> Out10/1
  Subsystem/5(Out5) -> Out5/1
  Subsystem/1(Out1) -> Out1/1
  Subsystem/7(Out7) -> Out7/1
  Subsystem/8(Out8) -> Out8/1
  Subsystem/3(Out3) -> Out3/1
  Subsystem/2(Out2) -> Out2/1
  Subsystem/16(Out16) -> Out16/1
  Subsystem/9(Out9) -> Out9/1
  Subsystem/12(Out12) -> Out12/1
  Subsystem/15(Out15) -> Out15/1
  Subsystem/4(Out4) -> Out4/1
  Subsystem/11(Out11) -> Out11/1
  In1/1 -> Subsystem8/1(In1)
  In3/1 -> Subsystem8/3(In3)
  In2/1 -> Subsystem8/2(In2)
  In4/1 -> Subsystem8/4(In4)
  In5/1 -> Subsystem8/5(In5)
  In7/1 -> Subsystem8/7(In7)
  In6/1 -> Subsystem8/6(In6)
  In9/1 -> Subsystem8/9(In9)
  In8/1 -> Subsystem8/8(In8)
  In12/1 -> Subsystem8/12(In12)
  In10/1 -> Subsystem8/10(In10)
  In11/1 -> Subsystem8/11(In11)
  In14/1 -> Subsystem8/14(In14)
  In13/1 -> Subsystem8/13(In13)
  In15/1 -> Subsystem8/15(In15)
  In16/1 -> Subsystem8/16(In16)
  Subsystem8/1(Out1) -> Subsystem/1(In1)
  Subsystem8/2(Out2) -> Subsystem/2(In2)
  Subsystem8/4(Out4) -> Subsystem/4(In4)
  Subsystem8/3(Out3) -> Subsystem/3(In3)
  Subsystem8/6(Out6) -> Subsystem/6(In6)
  Subsystem8/5(Out5) -> Subsystem/5(In5)
  Subsystem8/8(Out8) -> Subsystem/8(In8)
  Subsystem8/7(Out7) -> Subsystem/7(In7)
  Subsystem8/10(Out10) -> Subsystem/10(In10)
  Subsystem8/9(Out9) -> Subsystem/9(In9)
  Subsystem8/11(Out11) -> Subsystem/11(In11)
  Subsystem8/12(Out12) -> Subsystem/12(In12)
  Subsystem8/13(Out13) -> Subsystem/13(In13)
  Subsystem8/15(Out15) -> Subsystem/15(In15)
  Subsystem8/14(Out14) -> Subsystem/14(In14)
  Subsystem8/16(Out16) -> Subsystem/16(In16)
  In17/1 -> Key1/1(In1)
  In19/1 -> Key1/3(In3)
  In18/1 -> Key1/2(In2)
  In21/1 -> Key1/5(In5)
  In20/1 -> Key1/4(In4)
  In23/1 -> Key1/7(In7)
  In22/1 -> Key1/6(In6)
  In25/1 -> Key1/9(In9)
  In24/1 -> Key1/8(In8)
  In27/1 -> Key1/11(In11)
  In26/1 -> Key1/10(In10)
  In29/1 -> Key1/13(In13)
  In28/1 -> Key1/12(In12)
  In30/1 -> Key1/14(In14)
  In31/1 -> Key1/15(In15)
  In32/1 -> Key1/16(In16)
  Key1/14(Out14) -> Out30/1, Subsystem/30(In30)
  Key1/6(Out6) -> Out22/1, Subsystem/22(In22)
  Key1/13(Out13) -> Out29/1, Subsystem/29(In29)
  Key1/10(Out10) -> Out26/1, Subsystem/26(In26)
  Key1/5(Out5) -> Out21/1, Subsystem/21(In21)
  Key1/1(Out1) -> Out17/1, Subsystem/17(In17)
  Key1/7(Out7) -> Out23/1, Subsystem/23(In23)
  Key1/8(Out8) -> Out24/1, Subsystem/24(In24)
  Key1/3(Out3) -> Out19/1, Subsystem/19(In19)
  Key1/2(Out2) -> Out18/1, Subsystem/18(In18)
  Key1/16(Out16) -> Out32/1, Subsystem/32(In32)
  Key1/9(Out9) -> Out25/1, Subsystem/25(In25)
  Key1/12(Out12) -> Out28/1, Subsystem/28(In28)
  Key1/15(Out15) -> Out31/1, Subsystem/31(In31)
  Key1/4(Out4) -> Out20/1, Subsystem/20(In20)
  Key1/11(Out11) -> Out27/1, Subsystem/27(In27)

== system parallel/AES1 /Round11 ==
  In1 : Inport
  In2 : Inport  Port=2
  In3 : Inport  Port=3
  In4 : Inport  Port=4
  In5 : Inport  Port=5
  In6 : Inport  Port=6
  In7 : Inport  Port=7
  In8 : Inport  Port=8
  In9 : Inport  Port=9
  In10 : Inport  Port=10
  In11 : Inport  Port=11
  In12 : Inport  Port=12
  In13 : Inport  Port=13
  In14 : Inport  Port=14
  In15 : Inport  Port=15
  In16 : Inport  Port=16
  In17 : Inport  Port=17
  In18 : Inport  Port=18
  In19 : Inport  Port=19
  In20 : Inport  Port=20
  In21 : Inport  Port=21
  In22 : Inport  Port=22
  In23 : Inport  Port=23
  In24 : Inport  Port=24
  In25 : Inport  Port=25
  In26 : Inport  Port=26
  In27 : Inport  Port=27
  In28 : Inport  Port=28
  In29 : Inport  Port=29
  In30 : Inport  Port=30
  In31 : Inport  Port=31
  In32 : Inport  Port=32
  Subsystem : Subsystem
  Subsystem8 : Subsystem
  Out1 : Outport
  Out2 : Outport  Port=2
  Out3 : Outport  Port=3
  Out4 : Outport  Port=4
  Out5 : Outport  Port=5
  Out6 : Outport  Port=6
  Out7 : Outport  Port=7
  Out8 : Outport  Port=8
  Out9 : Outport  Port=9
  Out10 : Outport  Port=10
  Out11 : Outport  Port=11
  Out12 : Outport  Port=12
  Out13 : Outport  Port=13
  Out14 : Outport  Port=14
  Out15 : Outport  Port=15
  Out16 : Outport  Port=16
  wires:
  Subsystem/14(Out14) -> Out14/1
  Subsystem/6(Out6) -> Out6/1
  Subsystem/13(Out13) -> Out13/1
  Subsystem/10(Out10) -> Out10/1
  Subsystem/5(Out5) -> Out5/1
  Subsystem/1(Out1) -> Out1/1
  Subsystem/7(Out7) -> Out7/1
  Subsystem/8(Out8) -> Out8/1
  Subsystem/3(Out3) -> Out3/1
  Subsystem/2(Out2) -> Out2/1
  Subsystem/16(Out16) -> Out16/1
  Subsystem/9(Out9) -> Out9/1
  Subsystem/12(Out12) -> Out12/1
  Subsystem/15(Out15) -> Out15/1
  Subsystem/4(Out4) -> Out4/1
  Subsystem/11(Out11) -> Out11/1
  In1/1 -> Subsystem8/1(In1)
  In3/1 -> Subsystem8/3(In3)
  In2/1 -> Subsystem8/2(In2)
  In4/1 -> Subsystem8/4(In4)
  In5/1 -> Subsystem8/5(In5)
  In7/1 -> Subsystem8/7(In7)
  In6/1 -> Subsystem8/6(In6)
  In9/1 -> Subsystem8/9(In9)
  In8/1 -> Subsystem8/8(In8)
  In12/1 -> Subsystem8/12(In12)
  In10/1 -> Subsystem8/10(In10)
  In11/1 -> Subsystem8/11(In11)
  In14/1 -> Subsystem8/14(In14)
  In13/1 -> Subsystem8/13(In13)
  In15/1 -> Subsystem8/15(In15)
  In16/1 -> Subsystem8/16(In16)
  Subsystem8/1(Out1) -> Subsystem/1(In1)
  Subsystem8/2(Out2) -> Subsystem/2(In2)
  Subsystem8/4(Out4) -> Subsystem/4(In4)
  Subsystem8/3(Out3) -> Subsystem/3(In3)
  Subsystem8/6(Out6) -> Subsystem/6(In6)
  Subsystem8/5(Out5) -> Subsystem/5(In5)
  Subsystem8/8(Out8) -> Subsystem/8(In8)
  Subsystem8/7(Out7) -> Subsystem/7(In7)
  Subsystem8/10(Out10) -> Subsystem/10(In10)
  Subsystem8/9(Out9) -> Subsystem/9(In9)
  Subsystem8/11(Out11) -> Subsystem/11(In11)
  Subsystem8/12(Out12) -> Subsystem/12(In12)
  Subsystem8/13(Out13) -> Subsystem/13(In13)
  Subsystem8/15(Out15) -> Subsystem/15(In15)
  Subsystem8/14(Out14) -> Subsystem/14(In14)
  Subsystem8/16(Out16) -> Subsystem/16(In16)
  In31/1 -> Subsystem/31(In31)
  In24/1 -> Subsystem/24(In24)
  In23/1 -> Subsystem/23(In23)
  In22/1 -> Subsystem/22(In22)
  In20/1 -> Subsystem/20(In20)
  In21/1 -> Subsystem/21(In21)
  In25/1 -> Subsystem/25(In25)
  In26/1 -> Subsystem/26(In26)
  In27/1 -> Subsystem/27(In27)
  In28/1 -> Subsystem/28(In28)
  In29/1 -> Subsystem/29(In29)
  In30/1 -> Subsystem/30(In30)
  In32/1 -> Subsystem/32(In32)
  In17/1 -> Subsystem/17(In17)
  In18/1 -> Subsystem/18(In18)
  In19/1 -> Subsystem/19(In19)

== system parallel/AES1 /Round12 ==
  In1 : Inport
  In2 : Inport  Port=2
  In3 : Inport  Port=3
  In4 : Inport  Port=4
  In5 : Inport  Port=5
  In6 : Inport  Port=6
  In7 : Inport  Port=7
  In8 : Inport  Port=8
  In9 : Inport  Port=9
  In10 : Inport  Port=10
  In11 : Inport  Port=11
  In12 : Inport  Port=12
  In13 : Inport  Port=13
  In14 : Inport  Port=14
  In15 : Inport  Port=15
  In16 : Inport  Port=16
  In17 : Inport  Port=17
  In18 : Inport  Port=18
  In19 : Inport  Port=19
  In20 : Inport  Port=20
  In21 : Inport  Port=21
  In22 : Inport  Port=22
  In23 : Inport  Port=23
  In24 : Inport  Port=24
  In25 : Inport  Port=25
  In26 : Inport  Port=26
  In27 : Inport  Port=27
  In28 : Inport  Port=28
  In29 : Inport  Port=29
  In30 : Inport  Port=30
  In31 : Inport  Port=31
  In32 : Inport  Port=32
  Subsystem : Subsystem
  Subsystem8 : Subsystem
  Out1 : Outport
  Out2 : Outport  Port=2
  Out3 : Outport  Port=3
  Out4 : Outport  Port=4
  Out5 : Outport  Port=5
  Out6 : Outport  Port=6
  Out7 : Outport  Port=7
  Out8 : Outport  Port=8
  Out9 : Outport  Port=9
  Out10 : Outport  Port=10
  Out11 : Outport  Port=11
  Out12 : Outport  Port=12
  Out13 : Outport  Port=13
  Out14 : Outport  Port=14
  Out15 : Outport  Port=15
  Out16 : Outport  Port=16
  wires:
  Subsystem/14(Out14) -> Out14/1
  Subsystem/6(Out6) -> Out6/1
  Subsystem/13(Out13) -> Out13/1
  Subsystem/10(Out10) -> Out10/1
  Subsystem/5(Out5) -> Out5/1
  Subsystem/1(Out1) -> Out1/1
  Subsystem/7(Out7) -> Out7/1
  Subsystem/8(Out8) -> Out8/1
  Subsystem/3(Out3) -> Out3/1
  Subsystem/2(Out2) -> Out2/1
  Subsystem/16(Out16) -> Out16/1
  Subsystem/9(Out9) -> Out9/1
  Subsystem/12(Out12) -> Out12/1
  Subsystem/15(Out15) -> Out15/1
  Subsystem/4(Out4) -> Out4/1
  Subsystem/11(Out11) -> Out11/1
  In1/1 -> Subsystem8/1(In1)
  In3/1 -> Subsystem8/3(In3)
  In2/1 -> Subsystem8/2(In2)
  In4/1 -> Subsystem8/4(In4)
  In5/1 -> Subsystem8/5(In5)
  In7/1 -> Subsystem8/7(In7)
  In6/1 -> Subsystem8/6(In6)
  In9/1 -> Subsystem8/9(In9)
  In8/1 -> Subsystem8/8(In8)
  In12/1 -> Subsystem8/12(In12)
  In10/1 -> Subsystem8/10(In10)
  In11/1 -> Subsystem8/11(In11)
  In14/1 -> Subsystem8/14(In14)
  In13/1 -> Subsystem8/13(In13)
  In15/1 -> Subsystem8/15(In15)
  In16/1 -> Subsystem8/16(In16)
  Subsystem8/1(Out1) -> Subsystem/1(In1)
  Subsystem8/2(Out2) -> Subsystem/2(In2)
  Subsystem8/4(Out4) -> Subsystem/4(In4)
  Subsystem8/3(Out3) -> Subsystem/3(In3)
  Subsystem8/6(Out6) -> Subsystem/6(In6)
  Subsystem8/5(Out5) -> Subsystem/5(In5)
  Subsystem8/8(Out8) -> Subsystem/8(In8)
  Subsystem8/7(Out7) -> Subsystem/7(In7)
  Subsystem8/10(Out10) -> Subsystem/10(In10)
  Subsystem8/9(Out9) -> Subsystem/9(In9)
  Subsystem8/11(Out11) -> Subsystem/11(In11)
  Subsystem8/12(Out12) -> Subsystem/12(In12)
  Subsystem8/13(Out13) -> Subsystem/13(In13)
  Subsystem8/15(Out15) -> Subsystem/15(In15)
  Subsystem8/14(Out14) -> Subsystem/14(In14)
  Subsystem8/16(Out16) -> Subsystem/16(In16)
  In31/1 -> Subsystem/31(In31)
  In24/1 -> Subsystem/24(In24)
  In23/1 -> Subsystem/23(In23)
  In22/1 -> Subsystem/22(In22)
  In20/1 -> Subsystem/20(In20)
  In21/1 -> Subsystem/21(In21)
  In25/1 -> Subsystem/25(In25)
  In26/1 -> Subsystem/26(In26)
  In27/1 -> Subsystem/27(In27)
  In28/1 -> Subsystem/28(In28)
  In29/1 -> Subsystem/29(In29)
  In30/1 -> Subsystem/30(In30)
  In32/1 -> Subsystem/32(In32)
  In17/1 -> Subsystem/17(In17)
  In18/1 -> Subsystem/18(In18)
  In19/1 -> Subsystem/19(In19)

== system parallel/AES1 /Round13 ==
  In1 : Inport
  In2 : Inport  Port=2
  In3 : Inport  Port=3
  In4 : Inport  Port=4
  In5 : Inport  Port=5
  In6 : Inport  Port=6
  In7 : Inport  Port=7
  In8 : Inport  Port=8
  In9 : Inport  Port=9
  In10 : Inport  Port=10
  In11 : Inport  Port=11
  In12 : Inport  Port=12
  In13 : Inport  Port=13
  In14 : Inport  Port=14
  In15 : Inport  Port=15
  In16 : Inport  Port=16
  In17 : Inport  Port=17
  In18 : Inport  Port=18
  In19 : Inport  Port=19
  In20 : Inport  Port=20
  In21 : Inport  Port=21
  In22 : Inport  Port=22
  In23 : Inport  Port=23
  In24 : Inport  Port=24
  In25 : Inport  Port=25
  In26 : Inport  Port=26
  In27 : Inport  Port=27
  In28 : Inport  Port=28
  In29 : Inport  Port=29
  In30 : Inport  Port=30
  In31 : Inport  Port=31
  In32 : Inport  Port=32
  Subsystem : Subsystem
  Subsystem8 : Subsystem
  Out1 : Outport
  Out2 : Outport  Port=2
  Out3 : Outport  Port=3
  Out4 : Outport  Port=4
  Out5 : Outport  Port=5
  Out6 : Outport  Port=6
  Out7 : Outport  Port=7
  Out8 : Outport  Port=8
  Out9 : Outport  Port=9
  Out10 : Outport  Port=10
  Out11 : Outport  Port=11
  Out12 : Outport  Port=12
  Out13 : Outport  Port=13
  Out14 : Outport  Port=14
  Out15 : Outport  Port=15
  Out16 : Outport  Port=16
  wires:
  Subsystem/14(Out14) -> Out14/1
  Subsystem/6(Out6) -> Out6/1
  Subsystem/13(Out13) -> Out13/1
  Subsystem/10(Out10) -> Out10/1
  Subsystem/5(Out5) -> Out5/1
  Subsystem/1(Out1) -> Out1/1
  Subsystem/7(Out7) -> Out7/1
  Subsystem/8(Out8) -> Out8/1
  Subsystem/3(Out3) -> Out3/1
  Subsystem/2(Out2) -> Out2/1
  Subsystem/16(Out16) -> Out16/1
  Subsystem/9(Out9) -> Out9/1
  Subsystem/12(Out12) -> Out12/1
  Subsystem/15(Out15) -> Out15/1
  Subsystem/4(Out4) -> Out4/1
  Subsystem/11(Out11) -> Out11/1
  In1/1 -> Subsystem8/1(In1)
  In3/1 -> Subsystem8/3(In3)
  In2/1 -> Subsystem8/2(In2)
  In4/1 -> Subsystem8/4(In4)
  In5/1 -> Subsystem8/5(In5)
  In7/1 -> Subsystem8/7(In7)
  In6/1 -> Subsystem8/6(In6)
  In9/1 -> Subsystem8/9(In9)
  In8/1 -> Subsystem8/8(In8)
  In12/1 -> Subsystem8/12(In12)
  In10/1 -> Subsystem8/10(In10)
  In11/1 -> Subsystem8/11(In11)
  In14/1 -> Subsystem8/14(In14)
  In13/1 -> Subsystem8/13(In13)
  In15/1 -> Subsystem8/15(In15)
  In16/1 -> Subsystem8/16(In16)
  Subsystem8/1(Out1) -> Subsystem/1(In1)
  Subsystem8/2(Out2) -> Subsystem/2(In2)
  Subsystem8/4(Out4) -> Subsystem/4(In4)
  Subsystem8/3(Out3) -> Subsystem/3(In3)
  Subsystem8/6(Out6) -> Subsystem/6(In6)
  Subsystem8/5(Out5) -> Subsystem/5(In5)
  Subsystem8/8(Out8) -> Subsystem/8(In8)
  Subsystem8/7(Out7) -> Subsystem/7(In7)
  Subsystem8/10(Out10) -> Subsystem/10(In10)
  Subsystem8/9(Out9) -> Subsystem/9(In9)
  Subsystem8/11(Out11) -> Subsystem/11(In11)
  Subsystem8/12(Out12) -> Subsystem/12(In12)
  Subsystem8/13(Out13) -> Subsystem/13(In13)
  Subsystem8/15(Out15) -> Subsystem/15(In15)
  Subsystem8/14(Out14) -> Subsystem/14(In14)
  Subsystem8/16(Out16) -> Subsystem/16(In16)
  In31/1 -> Subsystem/31(In31)
  In24/1 -> Subsystem/24(In24)
  In23/1 -> Subsystem/23(In23)
  In22/1 -> Subsystem/22(In22)
  In20/1 -> Subsystem/20(In20)
  In21/1 -> Subsystem/21(In21)
  In25/1 -> Subsystem/25(In25)
  In26/1 -> Subsystem/26(In26)
  In27/1 -> Subsystem/27(In27)
  In28/1 -> Subsystem/28(In28)
  In29/1 -> Subsystem/29(In29)
  In30/1 -> Subsystem/30(In30)
  In32/1 -> Subsystem/32(In32)
  In17/1 -> Subsystem/17(In17)
  In18/1 -> Subsystem/18(In18)
  In19/1 -> Subsystem/19(In19)

== system parallel/AES1 /Round14 ==
  In1 : Inport
  In2 : Inport  Port=2
  In3 : Inport  Port=3
  In4 : Inport  Port=4
  In5 : Inport  Port=5
  In6 : Inport  Port=6
  In7 : Inport  Port=7
  In8 : Inport  Port=8
  In9 : Inport  Port=9
  In10 : Inport  Port=10
  In11 : Inport  Port=11
  In12 : Inport  Port=12
  In13 : Inport  Port=13
  In14 : Inport  Port=14
  In15 : Inport  Port=15
  In16 : Inport  Port=16
  In17 : Inport  Port=17
  In18 : Inport  Port=18
  In19 : Inport  Port=19
  In20 : Inport  Port=20
  In21 : Inport  Port=21
  In22 : Inport  Port=22
  In23 : Inport  Port=23
  In24 : Inport  Port=24
  In25 : Inport  Port=25
  In26 : Inport  Port=26
  In27 : Inport  Port=27
  In28 : Inport  Port=28
  In29 : Inport  Port=29
  In30 : Inport  Port=30
  In31 : Inport  Port=31
  In32 : Inport  Port=32
  Subsystem : Subsystem
  Subsystem8 : Subsystem
  Out1 : Outport
  Out2 : Outport  Port=2
  Out3 : Outport  Port=3
  Out4 : Outport  Port=4
  Out5 : Outport  Port=5
  Out6 : Outport  Port=6
  Out7 : Outport  Port=7
  Out8 : Outport  Port=8
  Out9 : Outport  Port=9
  Out10 : Outport  Port=10
  Out11 : Outport  Port=11
  Out12 : Outport  Port=12
  Out13 : Outport  Port=13
  Out14 : Outport  Port=14
  Out15 : Outport  Port=15
  Out16 : Outport  Port=16
  wires:
  Subsystem/14(Out14) -> Out14/1
  Subsystem/6(Out6) -> Out6/1
  Subsystem/13(Out13) -> Out13/1
  Subsystem/10(Out10) -> Out10/1
  Subsystem/5(Out5) -> Out5/1
  Subsystem/1(Out1) -> Out1/1
  Subsystem/7(Out7) -> Out7/1
  Subsystem/8(Out8) -> Out8/1
  Subsystem/3(Out3) -> Out3/1
  Subsystem/2(Out2) -> Out2/1
  Subsystem/16(Out16) -> Out16/1
  Subsystem/9(Out9) -> Out9/1
  Subsystem/12(Out12) -> Out12/1
  Subsystem/15(Out15) -> Out15/1
  Subsystem/4(Out4) -> Out4/1
  Subsystem/11(Out11) -> Out11/1
  In1/1 -> Subsystem8/1(In1)
  In3/1 -> Subsystem8/3(In3)
  In2/1 -> Subsystem8/2(In2)
  In4/1 -> Subsystem8/4(In4)
  In5/1 -> Subsystem8/5(In5)
  In7/1 -> Subsystem8/7(In7)
  In6/1 -> Subsystem8/6(In6)
  In9/1 -> Subsystem8/9(In9)
  In8/1 -> Subsystem8/8(In8)
  In12/1 -> Subsystem8/12(In12)
  In10/1 -> Subsystem8/10(In10)
  In11/1 -> Subsystem8/11(In11)
  In14/1 -> Subsystem8/14(In14)
  In13/1 -> Subsystem8/13(In13)
  In15/1 -> Subsystem8/15(In15)
  In16/1 -> Subsystem8/16(In16)
  Subsystem8/1(Out1) -> Subsystem/1(In1)
  Subsystem8/2(Out2) -> Subsystem/2(In2)
  Subsystem8/4(Out4) -> Subsystem/4(In4)
  Subsystem8/3(Out3) -> Subsystem/3(In3)
  Subsystem8/6(Out6) -> Subsystem/6(In6)
  Subsystem8/5(Out5) -> Subsystem/5(In5)
  Subsystem8/8(Out8) -> Subsystem/8(In8)
  Subsystem8/7(Out7) -> Subsystem/7(In7)
  Subsystem8/10(Out10) -> Subsystem/10(In10)
  Subsystem8/9(Out9) -> Subsystem/9(In9)
  Subsystem8/11(Out11) -> Subsystem/11(In11)
  Subsystem8/12(Out12) -> Subsystem/12(In12)
  Subsystem8/13(Out13) -> Subsystem/13(In13)
  Subsystem8/15(Out15) -> Subsystem/15(In15)
  Subsystem8/14(Out14) -> Subsystem/14(In14)
  Subsystem8/16(Out16) -> Subsystem/16(In16)
  In31/1 -> Subsystem/31(In31)
  In24/1 -> Subsystem/24(In24)
  In23/1 -> Subsystem/23(In23)
  In22/1 -> Subsystem/22(In22)
  In20/1 -> Subsystem/20(In20)
  In21/1 -> Subsystem/21(In21)
  In25/1 -> Subsystem/25(In25)
  In26/1 -> Subsystem/26(In26)
  In27/1 -> Subsystem/27(In27)
  In28/1 -> Subsystem/28(In28)
  In29/1 -> Subsystem/29(In29)
  In30/1 -> Subsystem/30(In30)
  In32/1 -> Subsystem/32(In32)
  In17/1 -> Subsystem/17(In17)
  In18/1 -> Subsystem/18(In18)
  In19/1 -> Subsystem/19(In19)
